simulink model "train_system_3Brakes"  (R2018b)
settings: Solver=VariableStepAuto  StartTime=1.0  StopTime=700.0  RelTol=1e-3
values from neighbouring files (symbols this model uses):
  brake_status = -1    [main.m]
  vmax = 28.5    [fsm_code.m]    (also in main.m)
  vmin = 20    [fsm_code.m]    (also in main.m)
settings Model: Creator=aniruddhgp  LastModifiedBy=aniruddhgp

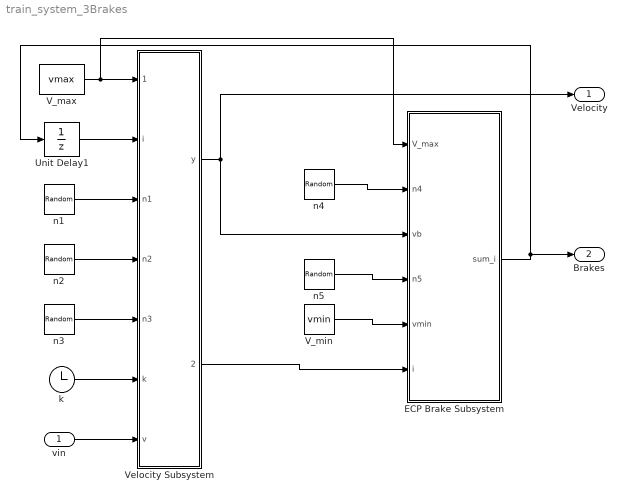
== system train_system_3Brakes ==
  vin : Inport
  ECP Brake Subsystem : Subsystem
  Unit Delay1 : UnitDelay  SampleTime=-1
  V_max : Constant  Value=vmax
  V_min : Constant  Value=vmin
  Velocity Subsystem : Stateflow chart  TreatAsAtomicUnit=on
  k : Clock
  n1 : RandomNumber  SampleTime=0.1
  n2 : RandomNumber  Variance=0.1  SampleTime=0.1
  n3 : RandomNumber  Variance=0.3  SampleTime=0.1
  n4 : RandomNumber  Variance=3  SampleTime=0.1
  n5 : RandomNumber  Variance=3  SampleTime=0.1
  Velocity : Outport
  Brakes : Outport  Port=2
  wires:
  n3/1 -> Velocity Subsystem/5(n3)
  n1/1 -> Velocity Subsystem/3(n1)
  V_max/1 -> Velocity Subsystem/1(vmax), ECP Brake Subsystem/1(V_max)
  n2/1 -> Velocity Subsystem/4(n2)
  k/1 -> Velocity Subsystem/6(k)
  Velocity Subsystem/1(y) -> Velocity/1, ECP Brake Subsystem/3(vb)
  Unit Delay1/1 -> Velocity Subsystem/2(i)
  Velocity Subsystem/2(i_vtob) -> ECP Brake Subsystem/6(i)
  ECP Brake Subsystem/1(sum_i) -> Brakes/1, Unit Delay1/1
  n4/1 -> ECP Brake Subsystem/2(n4)
  n5/1 -> ECP Brake Subsystem/4(n5)
  V_min/1 -> ECP Brake Subsystem/5(vmin)
  vin/1 -> Velocity Subsystem/7(v)

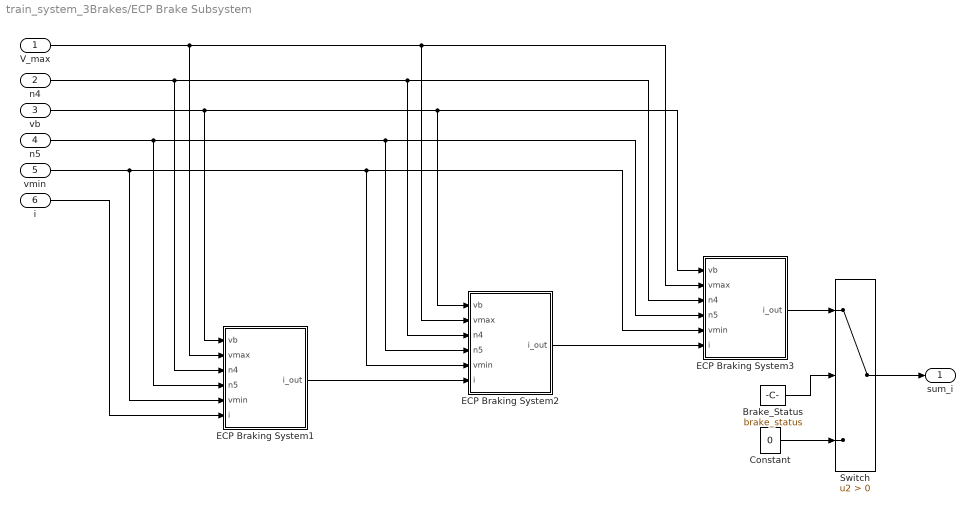
== system train_system_3Brakes/ECP Brake Subsystem ==
  V_max : Inport
  n4 : Inport  Port=2
  vb : Inport  Port=3
  n5 : Inport  Port=4
  vmin : Inport  Port=5
  i : Inport  Port=6
  Brake_Status : Constant  Value=brake_status
  Constant : Constant  Value=0
  ECP Braking System1 : Stateflow chart  TreatAsAtomicUnit=on
  ECP Braking System2 : Stateflow chart  TreatAsAtomicUnit=on
  ECP Braking System3 : Stateflow chart  TreatAsAtomicUnit=on
  Switch : Switch  Criteria=u2 > Threshold
  sum_i : Outport
  wires:
  ECP Braking System2/1(i_out) -> ECP Braking System3/6(i)
  ECP Braking System1/1(i_out) -> ECP Braking System2/6(i)
  V_max/1 -> ECP Braking System1/2(vmax), ECP Braking System2/2(vmax), ECP Braking System3/2(vmax)
  n4/1 -> ECP Braking System3/3(n4), ECP Braking System2/3(n4), ECP Braking System1/3(n4)
  vb/1 -> ECP Braking System1/1(vb), ECP Braking System2/1(vb), ECP Braking System3/1(vb)
  n5/1 -> ECP Braking System1/4(n5), ECP Braking System2/4(n5), ECP Braking System3/4(n5)
  vmin/1 -> ECP Braking System1/5(vmin), ECP Braking System2/5(vmin), ECP Braking System3/5(vmin)
  i/1 -> ECP Braking System1/6(i)
  ECP Braking System3/1(i_out) -> Switch/1
  Constant/1 -> Switch/3
  Switch/1 -> sum_i/1
  Brake_Status/1 -> Switch/2

== stateflow chart train_system_3Brakes/ECP Brake Subsystem/ECP Braking System1 ==
  state q1_5
    c1 = c1;
    c2 = c2;
    disp("Fail1");
  state q1_1
    c1 = n4;
    c2 = c2;
  state q1_2
    c1 = c1 + 1;
    c2 = c2;
    p = randi(1000) <= 1000;
  state q1_4
    c1 = c1;
    c2 = c2 + 1;
  state q1_3
    c1 = c1;
    c2 = n5;
  (default) -> q1_1
  q1_2 -> q1_5 [order 2] : [(c1 > 1) && (p == 0)]
  q1_1 -> q1_2 : [vb > vmax]{c1 = -abs(c1);}
  q1_2 -> q1_3 [order 1] : [(c1 > 1) && (p==1)]{i_out = i+1;}
  q1_4 -> q1_1 : [c2 > 1]{i_out = i-1;}
  q1_3 -> q1_4 : [vb < vmin]{c2 = -abs(c2);}
  data: vb input; vmax input; n4 input; n5 input; vmin input; c1 local =0; c2 local =0; i_out output; i input =0; p local

== stateflow chart train_system_3Brakes/ECP Brake Subsystem/ECP Braking System2 ==
  state q1_1
    c1 = n4;
    c2 = c2;
  state q1_2
    c1 = c1 + 1;
    c2 = c2;
    p = randi(1000) <= 1000;
  state q1_5
    c1 = c1;
    c2 = c2;
    disp("Fail2");
  state q1_4
    c1 = c1;
    c2 = c2 + 1;
  state q1_3
    c1 = c1;
    c2 = n5;
  (default) -> q1_1
  q1_1 -> q1_2 : [vb > vmax]{c1 = -abs(c1);}
  q1_2 -> q1_5 [order 2] : [(c1 > 1) && (p==0)]
  q1_2 -> q1_3 [order 1] : [(c1 > 1) && (p==1)]{i_out = i+1;}
  q1_4 -> q1_1 : [c2 > 1]{i_out = i-1;}
  q1_3 -> q1_4 : [vb < vmin]{c2 = -abs(c2);}
  data: vb input; vmax input; n4 input; n5 input; vmin input; c1 local =0; c2 local =0; i_out output; i input =0; p local

== stateflow chart train_system_3Brakes/Velocity Subsystem ==
  state qv_2
    next = prev-0.5*max(0,i-1)+n2;
    y = next + n3; prev = y;
    i_vtob = i;
  state qv_1
    prev = v;
    next = 0.1353*prev+0.8647*[25+2.5*sin(k)]+n1;
    y = next + n3; prev = y;
    i_vtob = i;
  state qv_3
    next = prev-0.5*max(0,i-1)+n3;
    y = next + n3; prev = y;
    i_vtob = i;
  (default) -> qv_1
  qv_1 -> qv_2 : [y > vmax]
  qv_2 -> qv_3 : [i > 0]
  qv_3 -> qv_1 : [i == 0]
  data: y output =0; vmax input; i input; n1 input; n2 input; n3 input; k input; next local; i_vtob output =0; v input; prev local

== stateflow chart train_system_3Brakes/ECP Brake Subsystem/ECP Braking System3 ==
  state q1_1
    c1 = n4;
    c2 = c2;
  state q1_2
    c1 = c1 + 1;
    c2 = c2;
    p = randi(1000) <= 1000;
  state q1_5
    c1 = c1;
    c2 = c2;
    disp("Fail6");
  state q1_4
    c1 = c1;
    c2 = c2 + 1;
  state q1_3
    c1 = c1;
    c2 = n5;
  (default) -> q1_1
  q1_1 -> q1_2 : [vb > vmax]{c1 = -abs(c1);}
  q1_2 -> q1_5 [order 2] : [(c1 > 1) && (p==0)]
  q1_4 -> q1_1 : [c2 > 1]{i_out = i-1;}
  q1_2 -> q1_3 [order 1] : [(c1 > 1) && (p==1)]{i_out = i+1;}
  q1_3 -> q1_4 : [vb < vmin]{c2 = -abs(c2);}
  data: vb input; vmax input; n4 input; n5 input; vmin input; c1 local =0; c2 local =0; i_out output; i input =0; p local
